simulink subsystem "SlipRateClc"  (R2021b)
settings: Solver=VariableStepAuto  StartTime=0.0  StopTime=10.0  RelTol=1e-3
settings Model: Creator=tsuyoshi  LastModifiedBy=tsuyoshi

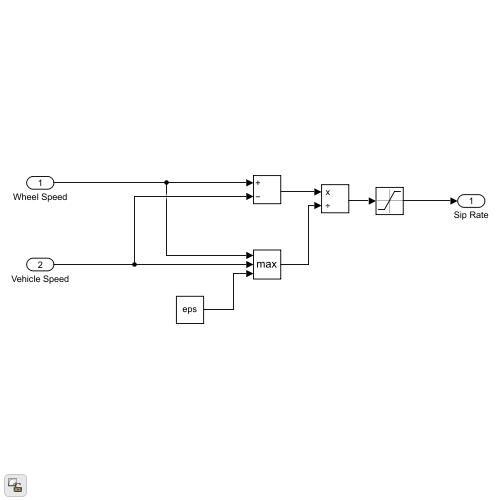
[thumbnail: Simulink's stored preview of the top-level diagram]
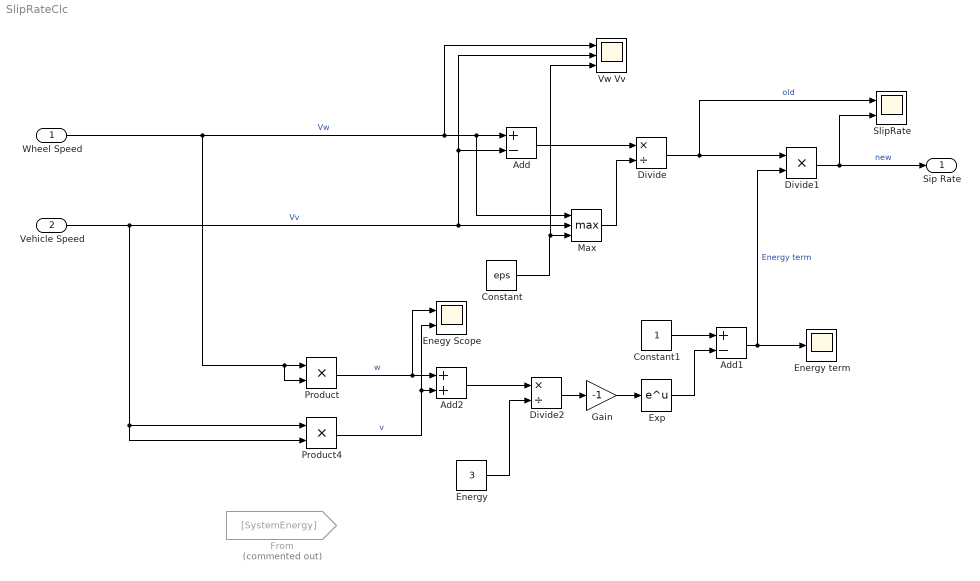
== system SlipRateClc ==
  Wheel Speed : Inport
  Vehicle Speed : Inport  Port=2
  Add : Sum  Inputs=+-
  Add1 : Sum  Inputs=+-
  Add2 : Sum
  Constant : Constant  Value=eps
  Constant1 : Constant
  Divide : Product  Inputs=*/
  Divide1 : Product  Inputs=**
  Divide2 : Product  Inputs=*/
  Enegy Scope : Scope  NumInputPorts=2
  Energy : Constant  Value=3
  Energy term : Scope
  Exp : Math  SaturateOnIntegerOverflow=on
  From : From  Commented=on  GotoTag=SystemEnergy  TagVisibility=global
  Gain : Gain  Gain=-1
  Max : MinMax  Function=max  Inputs=3
  Product : Product
  Product4 : Product
  SlipRate : Scope  NumInputPorts=2
  Vw Vv : Scope  NumInputPorts=3
  Sip Rate : Outport  VectorParamsAs1DForOutWhenUnconnected=off
  wires:
  Vehicle Speed/1 -> Product4/1, Product4/2, Vw Vv/2, Add/2, Max/2  "Vv"
  Constant/1 -> Max/3, Vw Vv/3
  Max/1 -> Divide/2
  Divide/1 -> Divide1/1, SlipRate/1  "old"
  Wheel Speed/1 -> Max/1, Add/1, Vw Vv/1, Product/2, Product/1  "Vw"
  Add/1 -> Divide/1
  Divide1/1 -> SlipRate/2, Sip Rate/1  "new"
  Gain/1 -> Exp/1
  Add2/1 -> Divide2/1
  Energy/1 -> Divide2/2
  Divide2/1 -> Gain/1
  Constant1/1 -> Add1/1
  Exp/1 -> Add1/2
  Add1/1 -> Divide1/2, Energy term/1  "Energy term"
  Product4/1 -> Enegy Scope/2, Add2/2  "v"
  Product/1 -> Add2/1, Enegy Scope/1  "w"
